simulink model "jsbsim_comm"  (R2015b)
settings: Solver=VariableStepAuto  StartTime=0.0  StopTime=inf  FixedStep=1  RelTol=1e-3
libraries: instrumentlib x1, dspnetwork x1
settings Model: Creator=kdemarco3  LastModifiedBy=kdemarco3

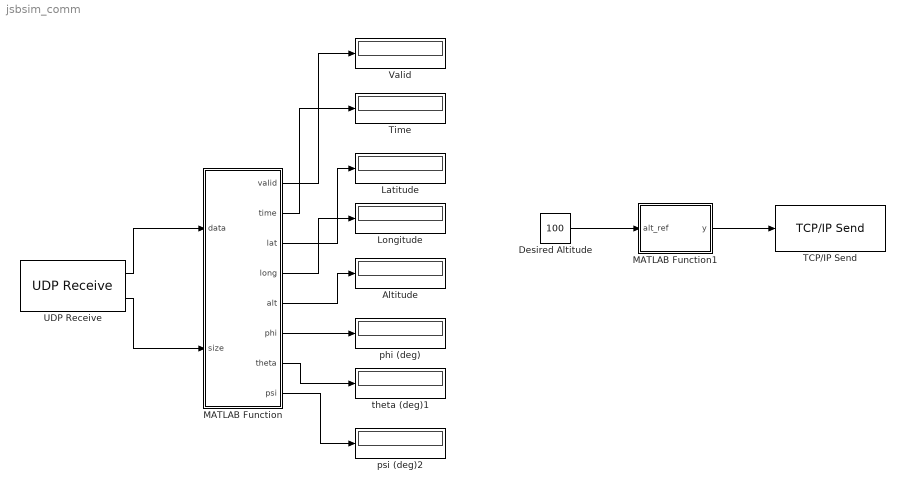
== system jsbsim_comm ==
  Altitude : Display
  Desired Altitude : Constant  Value=100
  Latitude : Display
  Longitude : Display
  MATLAB Function : MATLAB Function  TreatAsAtomicUnit=on
  MATLAB Function1 : MATLAB Function  TreatAsAtomicUnit=on
  TCP/IP Send : instrumentlib/TCP//IP Send  Host=localhost  Port=1137  EnableBlockingMode=off  Timeout=10  ByteOrder=BigEndian
  Time : Display
  UDP Receive : dspnetwork/UDP Receive  localURL='0.0.0.0'  localPort=6055  remoteURL='0.0.0.0'  remotePort=-1  recvBufferSize=8192  dims=512  signalDatatype=uint8  isVarSize=off  showBlockingTime=off  blockingTime=0  sampletime=0.1
  Valid : Display
  phi (deg) : Display
  psi (deg)2 : Display
  theta (deg)1 : Display
  wires:
  UDP Receive/1 -> MATLAB Function/1(data)
  UDP Receive/2 -> MATLAB Function/2(size)
  MATLAB Function/1(valid) -> Valid/1
  MATLAB Function/2(time) -> Time/1
  MATLAB Function/3(lat) -> Latitude/1
  MATLAB Function/4(long) -> Longitude/1
  MATLAB Function/6(phi) -> phi (deg)/1
  MATLAB Function/7(theta) -> theta (deg)1/1
  MATLAB Function/8(psi) -> psi (deg)2/1
  MATLAB Function/5(alt) -> Altitude/1
  MATLAB Function1/1(y) -> TCP/IP Send/1
  Desired Altitude/1 -> MATLAB Function1/1(alt_ref)

== matlab function jsbsim_comm/MATLAB Function1 ==
  data: alt_ref input; y output
function y = fcn(alt_ref)
%#codegen

alt_ref_cmd = 'set ap/altitude_setpoint ';
cmd_buf_size = length(alt_ref_cmd);

alt_ref_buf = zeros(1,64);
alt_ref_buf(1:length(alt_ref_cmd)) = alt_ref_cmd;

alt_ref_str = zeros(1,32);
coder.varsize('alt_ref_str');%, [1,32]);
coder.extrinsic('num2str'); 
alt_ref_str = num2str(alt_ref);

alt_ref_buf(length(alt_ref_cmd)+1:length(alt_ref_cmd)+length(alt_ref_str)) = alt_ref_str;

cmd_buf_size = cmd_buf_size + length(alt_ref_str);

%buffer = zeros(1,length(alt_ref_buf)+2);
buffer = zeros(1,256);

i = 1;
while i <= cmd_buf_size
    buffer(i) = alt_ref_buf(i);
    i = i + 1;
end
buffer(i) = 13;
i = i + 1;
buffer(i) = 10;

y = uint8(buffer);

% DEBUG CODE
%disp('----------------');
%coder.extrinsic('fprintf');
%loop = 1
%while loop <= i
%    fprintf('%d: %c %d \n', loop, y(loop), y(loop));
%    loop = loop + 1;
%end

== matlab function jsbsim_comm/MATLAB Function ==
  data: valid output; data input; time output; size input; lat output; long output; alt output; phi output; theta output; psi output
function [valid, time, lat, long, alt, phi, theta, psi]  = fcn(data,size)

valid = 0;
time = -1;
lat = -1;
long = -1;
phi = -1;
theta = -1;
psi = -1;
alt = -1;

%length(data)
% For debugging the received UDP message
%coder.extrinsic('cellstr'); 
%line = strtrim(strjoin(cellstr(char(data'))))

% Remove non-printable characters and spaces (32)
buffer = zeros(1,length(data));

i = 1; 
valid_chars = 1;
while (i <= length(data) && data(i) ~= 10)
    if data(i) > 32
        buffer(valid_chars) = data(i);
        valid_chars = valid_chars + 1;
    end
    i = i + 1;
end
valid_chars = valid_chars - 1;

numbers = NaN(1,100);
numbers_count = 1;
i = 1;
while i <= valid_chars
    %disp('Word');
    j = 0;
    str = '                                                                   ';
    while ( (j+1) <= length(str) && (i+j) <= length(buffer) && char(buffer(i+j)) ~= ',' && char(buffer(i+j)) ~= 0)
        %char(buffer(i+j))
        str(j+1) = char(buffer(i+j));
        j = j + 1;
    end
    
    number = real(str2double(str));
    
    if (~isnan(number))
        numbers(numbers_count) = number;
        numbers_count = numbers_count + 1;
    end
    
    i = i + j + 1;
end

numbers_count = numbers_count - 1;

if numbers_count == 20
    valid = 1;
end

% Map received numbers to outputs
time = numbers(1);
alt = numbers(13);
phi = numbers(14);
theta = numbers(15);
psi = numbers(16);
lat = numbers(19);
long = numbers(20);
